simulink model "ain"  (R2025a)
settings: Solver=VariableStepAuto  StartTime=0.0  StopTime=10.0  RelTol=1e-3
settings Model: Creator=matthewkeller  LastModifiedBy=matthewkeller

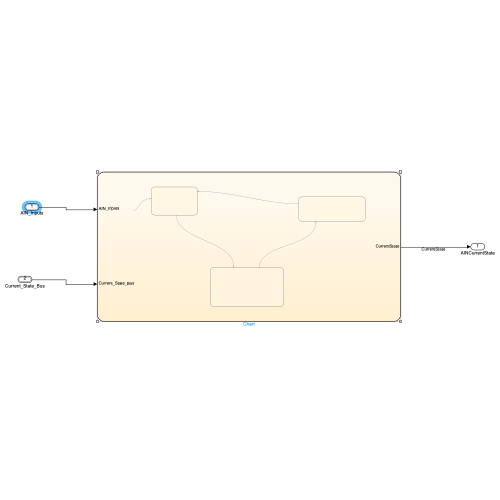
[thumbnail: Simulink's stored preview of the top-level diagram]
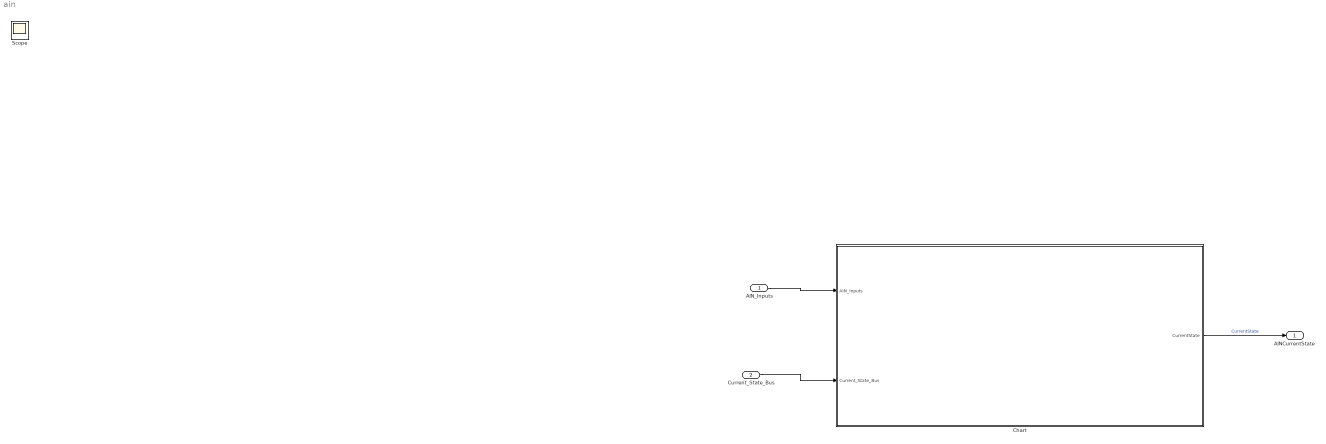
== system ain ==
  AIN_Inputs : Inport  OutDataTypeStr=Bus: AINStatusBus
  Current_State_Bus : Inport  Port=2  OutDataTypeStr=Bus: CurrentStateBus
  Chart : Stateflow chart  TreatAsAtomicUnit=on
  AINCurrentState : Outport
  Scope : Scope
      settings: ActiveDisplayYMinimum=-1  ActiveDisplayYMaximum=1
  wires:
  AIN_Inputs/1 -> Chart/1(AIN_Inputs)
  Chart/1(CurrentState) -> AINCurrentState/1  "CurrentState"
  Current_State_Bus/1 -> Chart/2(Current_State_Bus)

== stateflow chart ain/Chart ==
  settings: executeAtInitialization=1
  state AIN_Deactivated
    entry:
    CurrentState = StatusType.Deactivated;
  state AIN_Active
    entry:
    CurrentState = StatusType.Active;
  state AIN_Standby
    entry:
    CurrentState = StatusType.Standby;
  AIN_Active -> AIN_Deactivated : [AIN_Inputs.Cancel_AIN_Pressed]
  (default) -> AIN_Deactivated
  AIN_Deactivated -> AIN_Standby : [Current_State_Bus.ACCStatus == 2 && AIN_Inputs.V2X_Switch_ON && AIN_Inputs.Speed_LT_55_MPH]
  AIN_Standby -> AIN_Active : [AIN_Inputs.Activate_AIN_Pressed]
  data: AIN_Inputs input Bus: AINStatusBus; CurrentState output Enum: StatusType; Current_State_Bus input
